simulink model "problem3a_Group4"  (R2024b)
settings: Solver=VariableStepAuto  StartTime=0.0  StopTime=Sim_Time  RelTol=1e-3
undefined symbols (not defined in the file): l, L, R
settings Model: Creator=ASUS  LastModifiedBy=suave

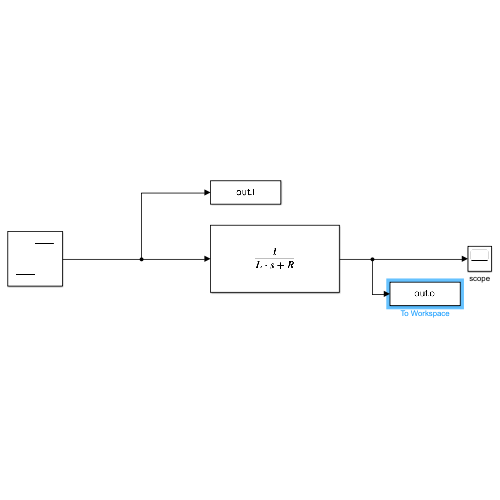
[thumbnail: Simulink's stored preview of the top-level diagram]
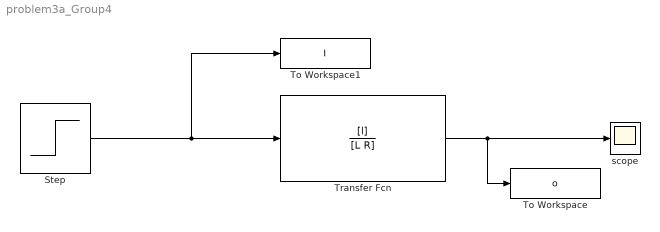
== system problem3a_Group4 ==
  Step : Step  SampleTime=0
  To Workspace : ToWorkspace  VariableName=o  SaveFormat=Timeseries  SampleTime=-1
  To Workspace1 : ToWorkspace  VariableName=I  SaveFormat=Timeseries  SampleTime=-1
  Transfer Fcn : TransferFcn  Numerator=[l]  Denominator=[L R]
  scope : Scope
  wires:
  Step/1 -> To Workspace1/1, Transfer Fcn/1
  Transfer Fcn/1 -> To Workspace/1, scope/1
